simulink model "Impedance_Gantry_Model_V8"  (R2021b)
settings: Solver=VariableStepAuto  StartTime=0  StopTime=5  FixedStep=0.001  RelTol=1e-3  AbsTol=1e-3  EnableMultiTasking=on
values from neighbouring files (symbols this model uses):
  Fmin = obj_x*obj_y*obj_z*obj_density*9.81/obj_coeff/obj_contactpt    (= 4.90500000153)    [Impedance_Control_V1.m]    (also in Impedance_Control_V2.m; Impedance_Control_V3.m; Impedance_Control_V4.m; Impedance_Control_V5.m)
  N = 100    [Gantry_Model_Sim_V1.m]    (also in Impedance_Control_V1.m = 10; Impedance_Control_V2.m = 10; Impedance_Control_V3.m = 40; Impedance_Control_V3_plot.m = 40)
  Ts = 0.01    [Gantry_Model_Sim_V1.m]    (also in Impedance_Control_V1.m = 0.0125; Impedance_Control_V2.m = 0.0125; Impedance_Control_V3.m = 0.0125; Impedance_Control_V4.m = 0.0125)
  z_clear = 1    [Impedance_Control_V1.m]    (also in Impedance_Control_V2.m; Impedance_Control_V3.m; Impedance_Control_V4.m; Impedance_Control_V5.m)
undefined symbols (not defined in the file or in its folder): X, Y, Z
libraries: sm_lib x89, nesl_utility x14, slpidlib x7
(part 4 of 4)

== system Impedance_Gantry_Model_V8/ObjectAndEnviroment/FBR ==
  FBR : sm_lib/Frames and Transforms/Rigid Transform  TranslationMethod=Cartesian  TranslationStandardOffset=0  TranslationLengthUnit=mm  TranslationStandardAxis=+Z  TranslationCartesianOffset=[0 0 0]  TranslationROffset=0  TranslationROffsetUnits=m  TranslationZOffset=0  TranslationZOffsetUnits=m  TranslationThetaOffset=0  TranslationThetaOffsetUnits=deg  RotationMethod=None  RotationAngleUnits=deg  RotationStandardAxis=+Z  RotationAngle=0.0  RotationArbitraryAxis=[0 0 1]  FollAlignAxisA=+X  BaseAlignAxisA=+Y  FollAlignAxisB=+Y  BaseAlignAxisB=+Z  RotationSequenceAxes=FollowerAxes  RotationSequence=XYX  RotationSequenceAngles=[0 0 0]  RotationSequenceAnglesUnits=deg  RotationMatrix=[1 0 0; 0 1 0; 0 0 1]
  FBRBall : sm_lib/Body Elements/Spherical Solid  GraphicAmbientColor=[0.15 0.15 0.15 1.0]  BasedOnType=Density  CenterOfMass=[0 0 0]  CenterOfMassUnits=m  GraphicDiffuseColor=[0.5 0.5 0.5]  Density=1000  DensityUnits=kg/m^3  DoExposeReferenceFrame=on  GraphicEmissiveColor=[0.0 0.0 0.0 1.0]  ExportEntireGeometry=on  SerializedExposedGeometries=<ExposedGeometries><ExposedGeometry><RawGeometryId>entire</RawGeometryId><ExposedGeometryId>G</ExposedGeometryId></ExposedGeometry></ExposedGeometries>  SerializedFrames=<Frames/>  MarkerShape=Sphere  MarkerSize=10  GraphicType=FromGeometry  InertiaType=CalculateFromGeometry  Mass=1  MassUnits=kg  MomentsOfInertia=[1 1 1]  MomentsOfInertiaUnits=kg*m^2  GraphicOpacity=1.0  ProductsOfInertia=[0 0 0]  ProductsOfInertiaUnits=kg*m^2  GraphicShininess=75  GraphicSpecularColor=[0.5 0.5 0.5 1.0]  SphereRadius=1  SphereRadiusUnits=mm  GraphicVisPropType=SimpleVisualProperties
  FBRConveyerDest : sm_lib/Forces and Torques/Spatial Contact Force  CoefficientOfDynamicFriction=0.5  CoefficientOfStaticFriction=0.5  SenseContactBaseRotation=off  SenseContactBaseTranslation=off  NormalDamping=30  NormalDampingUnits=N/(m/s)  SenseContactFollowerRotation=off  SenseContactFollowerTranslation=off  SenseContactSignal=off  NormalStiffness=1e4  NormalStiffnessUnits=N/m  FrictionalCriticalVelocity=1e-3  FrictionalCriticalVelocityUnits=m/s  ZeroCrossDetectContactStartAndEnd=off  FrictionType=SmoothStickSlip  SenseFrictionalForceMagnitude=off  SenseNormalForceMagnitude=off  NormalForceType=SmoothSpringDamper  SenseNormalVelocity=off  SenseSeparationDistance=off  SenseTangentialVelocity=off  SenseTangentialVelocityMagnitude=off  NormalTransitionRegionWidth=1e-5  NormalTransitionRegionWidthUnits=m
  FBRConveyerOri : sm_lib/Forces and Torques/Spatial Contact Force  CoefficientOfDynamicFriction=0.5  CoefficientOfStaticFriction=0.5  SenseContactBaseRotation=off  SenseContactBaseTranslation=off  NormalDamping=30  NormalDampingUnits=N/(m/s)  SenseContactFollowerRotation=off  SenseContactFollowerTranslation=off  SenseContactSignal=off  NormalStiffness=1e4  NormalStiffnessUnits=N/m  FrictionalCriticalVelocity=1e-3  FrictionalCriticalVelocityUnits=m/s  ZeroCrossDetectContactStartAndEnd=off  FrictionType=SmoothStickSlip  SenseFrictionalForceMagnitude=off  SenseNormalForceMagnitude=off  NormalForceType=SmoothSpringDamper  SenseNormalVelocity=off  SenseSeparationDistance=off  SenseTangentialVelocity=off  SenseTangentialVelocityMagnitude=off  NormalTransitionRegionWidth=1e-5  NormalTransitionRegionWidthUnits=m
  FBRGripper : sm_lib/Forces and Torques/Spatial Contact Force  CoefficientOfDynamicFriction=0.5  CoefficientOfStaticFriction=0.5  SenseContactBaseRotation=off  SenseContactBaseTranslation=off  NormalDamping=0  NormalDampingUnits=N/(m/s)  SenseContactFollowerRotation=off  SenseContactFollowerTranslation=off  SenseContactSignal=off  NormalStiffness=1e4  NormalStiffnessUnits=N/m  FrictionalCriticalVelocity=1e-3  FrictionalCriticalVelocityUnits=m/s  ZeroCrossDetectContactStartAndEnd=off  FrictionType=SmoothStickSlip  SenseFrictionalForceMagnitude=off  SenseNormalForceMagnitude=off  NormalForceType=SmoothSpringDamper  SenseNormalVelocity=off  SenseSeparationDistance=off  SenseTangentialVelocity=off  SenseTangentialVelocityMagnitude=off  NormalTransitionRegionWidth=1e-5  NormalTransitionRegionWidthUnits=m
  Obj : PMIOPort  Side=Left
  Gripper : PMIOPort  Port=2  Side=Right
  ConveyerOri : PMIOPort  Port=3  Side=Right
  ConveyerDest : PMIOPort  Port=4  Side=Right
  connections:
  ConveyerOri/RConn1 -- FBRConveyerOri/RConn1
  FBRBall/LConn1 -- FBRConveyerOri/LConn1 -- FBRConveyerDest/LConn1 -- FBRGripper/LConn1
  FBRBall/RConn1 -- FBR/RConn1
  Obj/RConn1 -- FBR/LConn1
  FBRConveyerDest/RConn1 -- ConveyerDest/RConn1
  Gripper/RConn1 -- FBRGripper/RConn1

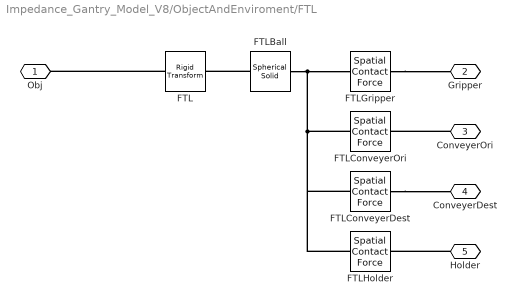
== system Impedance_Gantry_Model_V8/ObjectAndEnviroment/FTL ==
  FTL : sm_lib/Frames and Transforms/Rigid Transform  TranslationMethod=Cartesian  TranslationStandardOffset=0  TranslationLengthUnit=mm  TranslationStandardAxis=+Z  TranslationCartesianOffset=[0 25 30]  TranslationROffset=0  TranslationROffsetUnits=m  TranslationZOffset=0  TranslationZOffsetUnits=m  TranslationThetaOffset=0  TranslationThetaOffsetUnits=deg  RotationMethod=None  RotationAngleUnits=deg  RotationStandardAxis=+Z  RotationAngle=0.0  RotationArbitraryAxis=[0 0 1]  FollAlignAxisA=+X  BaseAlignAxisA=+Y  FollAlignAxisB=+Y  BaseAlignAxisB=+Z  RotationSequenceAxes=FollowerAxes  RotationSequence=XYX  RotationSequenceAngles=[0 0 0]  RotationSequenceAnglesUnits=deg  RotationMatrix=[1 0 0; 0 1 0; 0 0 1]
  FTLBall : sm_lib/Body Elements/Spherical Solid  GraphicAmbientColor=[0.15 0.15 0.15 1.0]  BasedOnType=Density  CenterOfMass=[0 0 0]  CenterOfMassUnits=m  GraphicDiffuseColor=[0.5 0.5 0.5]  Density=1000  DensityUnits=kg/m^3  DoExposeReferenceFrame=on  GraphicEmissiveColor=[0.0 0.0 0.0 1.0]  ExportEntireGeometry=on  SerializedExposedGeometries=<ExposedGeometries><ExposedGeometry><RawGeometryId>entire</RawGeometryId><ExposedGeometryId>G</ExposedGeometryId></ExposedGeometry></ExposedGeometries>  SerializedFrames=<Frames/>  MarkerShape=Sphere  MarkerSize=10  GraphicType=FromGeometry  InertiaType=CalculateFromGeometry  Mass=1  MassUnits=kg  MomentsOfInertia=[1 1 1]  MomentsOfInertiaUnits=kg*m^2  GraphicOpacity=1.0  ProductsOfInertia=[0 0 0]  ProductsOfInertiaUnits=kg*m^2  GraphicShininess=75  GraphicSpecularColor=[0.5 0.5 0.5 1.0]  SphereRadius=1  SphereRadiusUnits=mm  GraphicVisPropType=SimpleVisualProperties
  FTLConveyerDest : sm_lib/Forces and Torques/Spatial Contact Force  CoefficientOfDynamicFriction=0.5  CoefficientOfStaticFriction=0.5  SenseContactBaseRotation=off  SenseContactBaseTranslation=off  NormalDamping=30  NormalDampingUnits=N/(m/s)  SenseContactFollowerRotation=off  SenseContactFollowerTranslation=off  SenseContactSignal=off  NormalStiffness=1e4  NormalStiffnessUnits=N/m  FrictionalCriticalVelocity=1e-3  FrictionalCriticalVelocityUnits=m/s  ZeroCrossDetectContactStartAndEnd=off  FrictionType=SmoothStickSlip  SenseFrictionalForceMagnitude=off  SenseNormalForceMagnitude=off  NormalForceType=SmoothSpringDamper  SenseNormalVelocity=off  SenseSeparationDistance=off  SenseTangentialVelocity=off  SenseTangentialVelocityMagnitude=off  NormalTransitionRegionWidth=1e-5  NormalTransitionRegionWidthUnits=m
  FTLConveyerOri : sm_lib/Forces and Torques/Spatial Contact Force  CoefficientOfDynamicFriction=0.5  CoefficientOfStaticFriction=0.5  SenseContactBaseRotation=off  SenseContactBaseTranslation=off  NormalDamping=30  NormalDampingUnits=N/(m/s)  SenseContactFollowerRotation=off  SenseContactFollowerTranslation=off  SenseContactSignal=off  NormalStiffness=1e4  NormalStiffnessUnits=N/m  FrictionalCriticalVelocity=1e-3  FrictionalCriticalVelocityUnits=m/s  ZeroCrossDetectContactStartAndEnd=off  FrictionType=SmoothStickSlip  SenseFrictionalForceMagnitude=off  SenseNormalForceMagnitude=off  NormalForceType=SmoothSpringDamper  SenseNormalVelocity=off  SenseSeparationDistance=off  SenseTangentialVelocity=off  SenseTangentialVelocityMagnitude=off  NormalTransitionRegionWidth=1e-5  NormalTransitionRegionWidthUnits=m
  FTLGripper : sm_lib/Forces and Torques/Spatial Contact Force  CoefficientOfDynamicFriction=0.5  CoefficientOfStaticFriction=0.5  SenseContactBaseRotation=off  SenseContactBaseTranslation=off  NormalDamping=0  NormalDampingUnits=N/(m/s)  SenseContactFollowerRotation=off  SenseContactFollowerTranslation=off  SenseContactSignal=off  NormalStiffness=1e4  NormalStiffnessUnits=N/m  FrictionalCriticalVelocity=1e-3  FrictionalCriticalVelocityUnits=m/s  ZeroCrossDetectContactStartAndEnd=off  FrictionType=SmoothStickSlip  SenseFrictionalForceMagnitude=off  SenseNormalForceMagnitude=off  NormalForceType=SmoothSpringDamper  SenseNormalVelocity=off  SenseSeparationDistance=off  SenseTangentialVelocity=off  SenseTangentialVelocityMagnitude=off  NormalTransitionRegionWidth=1e-5  NormalTransitionRegionWidthUnits=m
  FTLHolder : sm_lib/Forces and Torques/Spatial Contact Force  CoefficientOfDynamicFriction=0.5  CoefficientOfStaticFriction=0.5  SenseContactBaseRotation=off  SenseContactBaseTranslation=off  NormalDamping=0  NormalDampingUnits=N/(m/s)  SenseContactFollowerRotation=off  SenseContactFollowerTranslation=off  SenseContactSignal=off  NormalStiffness=1e4  NormalStiffnessUnits=N/m  FrictionalCriticalVelocity=1e-3  FrictionalCriticalVelocityUnits=m/s  ZeroCrossDetectContactStartAndEnd=off  FrictionType=SmoothStickSlip  SenseFrictionalForceMagnitude=off  SenseNormalForceMagnitude=off  NormalForceType=SmoothSpringDamper  SenseNormalVelocity=off  SenseSeparationDistance=off  SenseTangentialVelocity=off  SenseTangentialVelocityMagnitude=off  NormalTransitionRegionWidth=1e-5  NormalTransitionRegionWidthUnits=m
  Obj : PMIOPort  Side=Left
  Gripper : PMIOPort  Port=2  Side=Right
  ConveyerOri : PMIOPort  Port=3  Side=Right
  ConveyerDest : PMIOPort  Port=4  Side=Right
  Holder : PMIOPort  Port=5  Side=Right
  connections:
  FTLBall/RConn1 -- FTL/RConn1
  FTLBall/LConn1 -- FTLConveyerDest/LConn1 -- FTLHolder/LConn1 -- FTLConveyerOri/LConn1 -- FTLGripper/LConn1
  FTLConveyerDest/RConn1 -- ConveyerDest/RConn1
  FTL/LConn1 -- Obj/RConn1
  FTLGripper/RConn1 -- Gripper/RConn1
  ConveyerOri/RConn1 -- FTLConveyerOri/RConn1
  Holder/RConn1 -- FTLHolder/RConn1

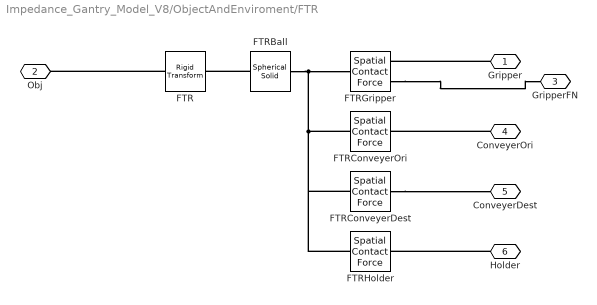
== system Impedance_Gantry_Model_V8/ObjectAndEnviroment/FTR ==
  FTR : sm_lib/Frames and Transforms/Rigid Transform  TranslationMethod=Cartesian  TranslationStandardOffset=0  TranslationLengthUnit=mm  TranslationStandardAxis=+Z  TranslationCartesianOffset=[0 0 30]  TranslationROffset=0  TranslationROffsetUnits=m  TranslationZOffset=0  TranslationZOffsetUnits=m  TranslationThetaOffset=0  TranslationThetaOffsetUnits=deg  RotationMethod=None  RotationAngleUnits=deg  RotationStandardAxis=+Z  RotationAngle=0.0  RotationArbitraryAxis=[0 0 1]  FollAlignAxisA=+X  BaseAlignAxisA=+Y  FollAlignAxisB=+Y  BaseAlignAxisB=+Z  RotationSequenceAxes=FollowerAxes  RotationSequence=XYX  RotationSequenceAngles=[0 0 0]  RotationSequenceAnglesUnits=deg  RotationMatrix=[1 0 0; 0 1 0; 0 0 1]
  FTRBall : sm_lib/Body Elements/Spherical Solid  GraphicAmbientColor=[0.15 0.15 0.15 1.0]  BasedOnType=Density  CenterOfMass=[0 0 0]  CenterOfMassUnits=m  GraphicDiffuseColor=[0.5 0.5 0.5]  Density=1000  DensityUnits=kg/m^3  DoExposeReferenceFrame=on  GraphicEmissiveColor=[0.0 0.0 0.0 1.0]  ExportEntireGeometry=on  SerializedExposedGeometries=<ExposedGeometries><ExposedGeometry><RawGeometryId>entire</RawGeometryId><ExposedGeometryId>G</ExposedGeometryId></ExposedGeometry></ExposedGeometries>  SerializedFrames=<Frames/>  MarkerShape=Sphere  MarkerSize=10  GraphicType=FromGeometry  InertiaType=CalculateFromGeometry  Mass=1  MassUnits=kg  MomentsOfInertia=[1 1 1]  MomentsOfInertiaUnits=kg*m^2  GraphicOpacity=1.0  ProductsOfInertia=[0 0 0]  ProductsOfInertiaUnits=kg*m^2  GraphicShininess=75  GraphicSpecularColor=[0.5 0.5 0.5 1.0]  SphereRadius=1  SphereRadiusUnits=mm  GraphicVisPropType=SimpleVisualProperties
  FTRConveyerDest : sm_lib/Forces and Torques/Spatial Contact Force  CoefficientOfDynamicFriction=0.5  CoefficientOfStaticFriction=0.5  SenseContactBaseRotation=off  SenseContactBaseTranslation=off  NormalDamping=30  NormalDampingUnits=N/(m/s)  SenseContactFollowerRotation=off  SenseContactFollowerTranslation=off  SenseContactSignal=off  NormalStiffness=1e4  NormalStiffnessUnits=N/m  FrictionalCriticalVelocity=1e-3  FrictionalCriticalVelocityUnits=m/s  ZeroCrossDetectContactStartAndEnd=off  FrictionType=SmoothStickSlip  SenseFrictionalForceMagnitude=off  SenseNormalForceMagnitude=off  NormalForceType=SmoothSpringDamper  SenseNormalVelocity=off  SenseSeparationDistance=off  SenseTangentialVelocity=off  SenseTangentialVelocityMagnitude=off  NormalTransitionRegionWidth=1e-5  NormalTransitionRegionWidthUnits=m
  FTRConveyerOri : sm_lib/Forces and Torques/Spatial Contact Force  CoefficientOfDynamicFriction=0.5  CoefficientOfStaticFriction=0.5  SenseContactBaseRotation=off  SenseContactBaseTranslation=off  NormalDamping=30  NormalDampingUnits=N/(m/s)  SenseContactFollowerRotation=off  SenseContactFollowerTranslation=off  SenseContactSignal=off  NormalStiffness=1e4  NormalStiffnessUnits=N/m  FrictionalCriticalVelocity=1e-3  FrictionalCriticalVelocityUnits=m/s  ZeroCrossDetectContactStartAndEnd=off  FrictionType=SmoothStickSlip  SenseFrictionalForceMagnitude=off  SenseNormalForceMagnitude=off  NormalForceType=SmoothSpringDamper  SenseNormalVelocity=off  SenseSeparationDistance=off  SenseTangentialVelocity=off  SenseTangentialVelocityMagnitude=off  NormalTransitionRegionWidth=1e-5  NormalTransitionRegionWidthUnits=m
  FTRGripper : sm_lib/Forces and Torques/Spatial Contact Force  CoefficientOfDynamicFriction=0.5  CoefficientOfStaticFriction=0.5  SenseContactBaseRotation=off  SenseContactBaseTranslation=off  NormalDamping=0  NormalDampingUnits=N/(m/s)  SenseContactFollowerRotation=off  SenseContactFollowerTranslation=off  SenseContactSignal=off  NormalStiffness=1e4  NormalStiffnessUnits=N/m  FrictionalCriticalVelocity=1e-3  FrictionalCriticalVelocityUnits=m/s  ZeroCrossDetectContactStartAndEnd=off  FrictionType=SmoothStickSlip  SenseFrictionalForceMagnitude=on  SenseNormalForceMagnitude=off  NormalForceType=SmoothSpringDamper  SenseNormalVelocity=off  SenseSeparationDistance=off  SenseTangentialVelocity=off  SenseTangentialVelocityMagnitude=off  NormalTransitionRegionWidth=1e-5  NormalTransitionRegionWidthUnits=m
  FTRHolder : sm_lib/Forces and Torques/Spatial Contact Force  CoefficientOfDynamicFriction=0.5  CoefficientOfStaticFriction=0.5  SenseContactBaseRotation=off  SenseContactBaseTranslation=off  NormalDamping=0  NormalDampingUnits=N/(m/s)  SenseContactFollowerRotation=off  SenseContactFollowerTranslation=off  SenseContactSignal=off  NormalStiffness=1e4  NormalStiffnessUnits=N/m  FrictionalCriticalVelocity=1e-3  FrictionalCriticalVelocityUnits=m/s  ZeroCrossDetectContactStartAndEnd=off  FrictionType=SmoothStickSlip  SenseFrictionalForceMagnitude=off  SenseNormalForceMagnitude=off  NormalForceType=SmoothSpringDamper  SenseNormalVelocity=off  SenseSeparationDistance=off  SenseTangentialVelocity=off  SenseTangentialVelocityMagnitude=off  NormalTransitionRegionWidth=1e-5  NormalTransitionRegionWidthUnits=m
  Gripper : PMIOPort  Side=Right
  Obj : PMIOPort  Port=2  Side=Left
  GripperFN : PMIOPort  Port=3  Side=Right
  ConveyerOri : PMIOPort  Port=4  Side=Right
  ConveyerDest : PMIOPort  Port=5  Side=Right
  Holder : PMIOPort  Port=6  Side=Right
  connections:
  FTRBall/LConn1 -- FTRConveyerDest/LConn1 -- FTRHolder/LConn1 -- FTRConveyerOri/LConn1 -- FTRGripper/LConn1
  FTRBall/RConn1 -- FTR/RConn1
  ConveyerOri/RConn1 -- FTRConveyerOri/RConn1
  FTR/LConn1 -- Obj/RConn1
  FTRConveyerDest/RConn1 -- ConveyerDest/RConn1
  Holder/RConn1 -- FTRHolder/RConn1
  Gripper/RConn1 -- FTRGripper/RConn1
  FTRGripper/RConn2 -- GripperFN/RConn1

== system Impedance_Gantry_Model_V8/Impedance Control/F desired logic/If Action Subsystem ==
  In1 : Inport
  Action Port : ActionPort  ActionPortLabel=if(u1 > 0 & u2 > 1 & u2 < 4)
  DesiredForce : Outport
  wires:
  In1/1 -> DesiredForce/1

== system Impedance_Gantry_Model_V8/Impedance Control/F desired logic/If Action Subsystem1 ==
  In1 : Inport
  Action Port : ActionPort  ActionPortLabel=else
  DesiredForce : Outport
  wires:
  In1/1 -> DesiredForce/1

== system Impedance_Gantry_Model_V8/Impedance Control/Left Grip desired logic/If Action Subsystem2 ==
  In1 : Inport
  Action Port : ActionPort  ActionPortLabel=if(u1 > 0)
  DesiredForce : Outport
  wires:
  In1/1 -> DesiredForce/1

== system Impedance_Gantry_Model_V8/Impedance Control/Left Grip desired logic/If Action Subsystem3 ==
  In1 : Inport
  Action Port : ActionPort  ActionPortLabel=else
  DesiredForce : Outport
  wires:
  In1/1 -> DesiredForce/1

== system Impedance_Gantry_Model_V8/Impedance Control/Right Grip desired logic/If Action Subsystem4 ==
  In1 : Inport
  Action Port : ActionPort  ActionPortLabel=if(u1 > 0)
  DesiredForce : Outport
  wires:
  In1/1 -> DesiredForce/1

== system Impedance_Gantry_Model_V8/Impedance Control/Right Grip desired logic/If Action Subsystem5 ==
  In1 : Inport
  Action Port : ActionPort  ActionPortLabel=else
  DesiredForce : Outport
  wires:
  In1/1 -> DesiredForce/1
